simulink model "decoder"  (R2025b)
settings: Solver=VariableStepAuto  StartTime=0.0  StopTime=10.0  RelTol=1e-3
settings Model: Creator=cyber  LastModifiedBy=cyber

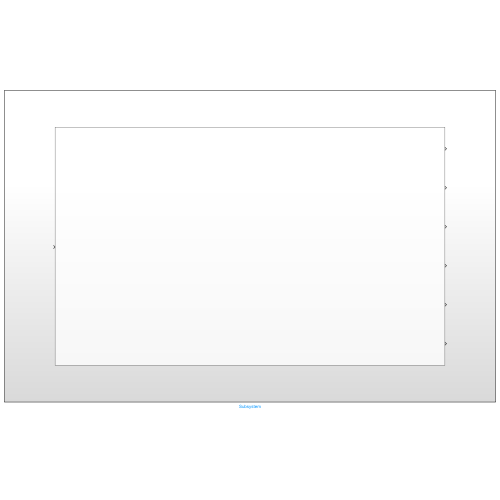
[thumbnail: Simulink's stored preview of the top-level diagram]
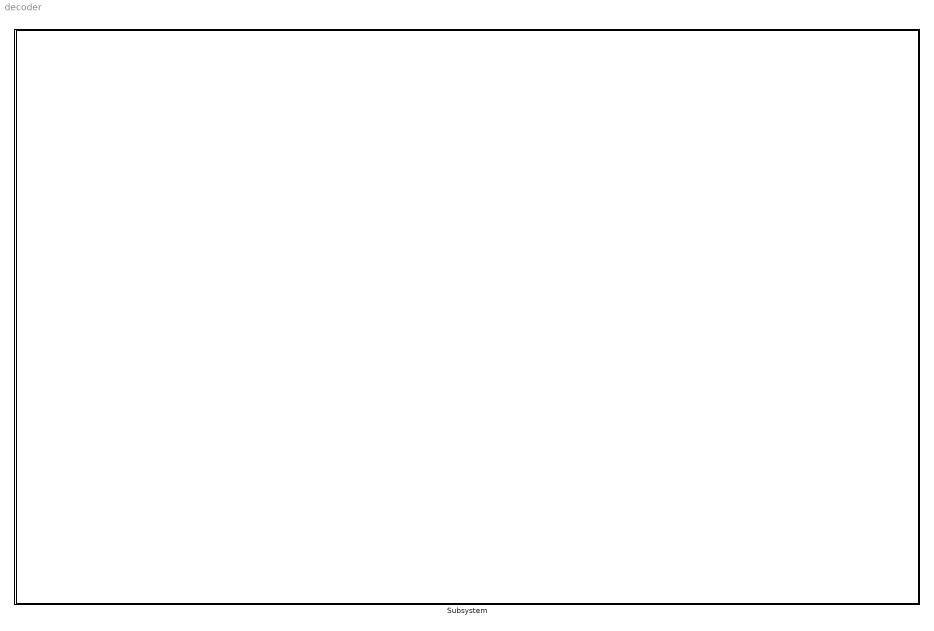
== system decoder ==
  Subsystem : Subsystem

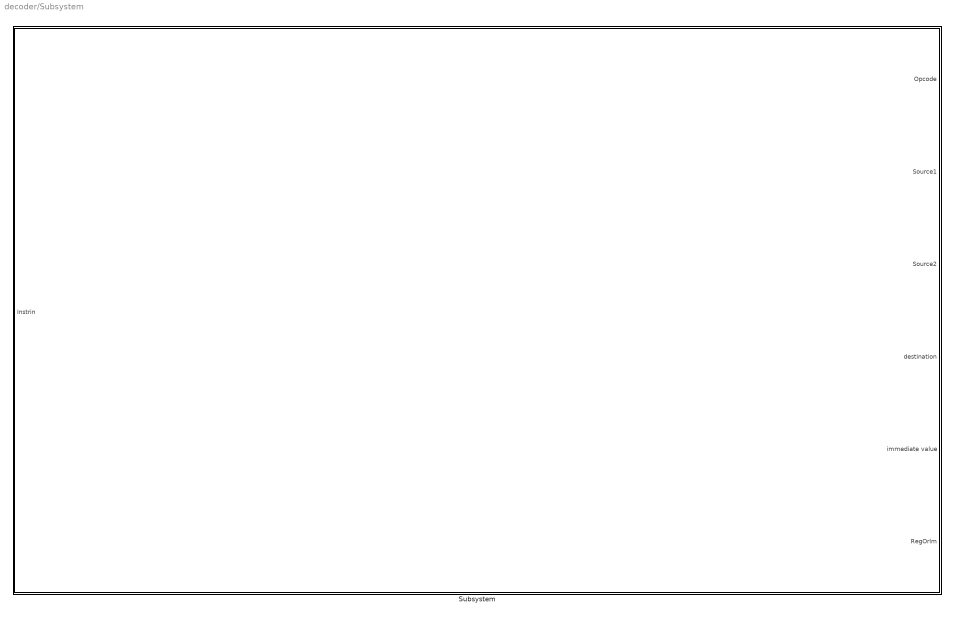
== system decoder/Subsystem ==
  Subsystem : Subsystem

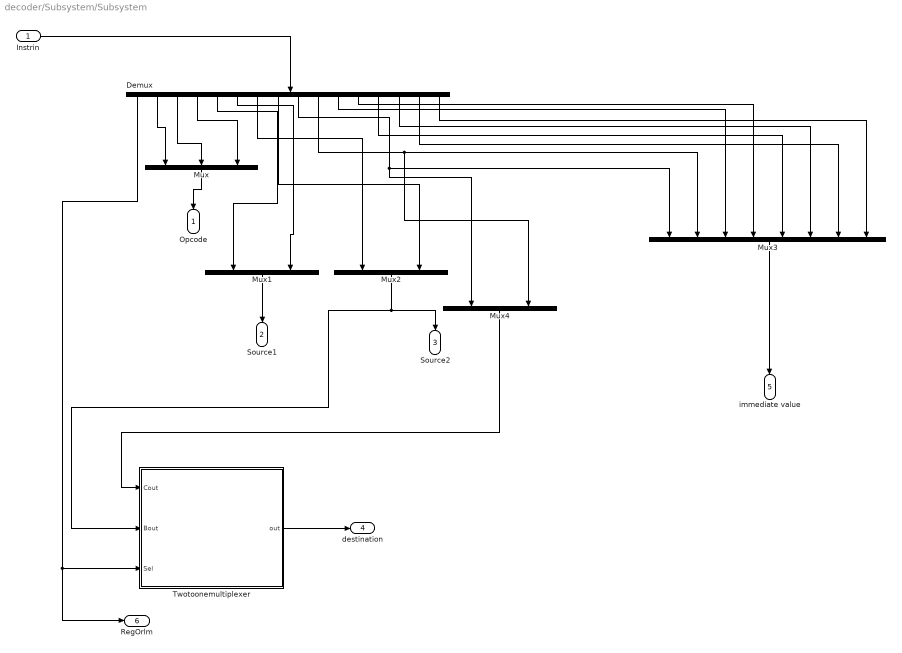
== system decoder/Subsystem/Subsystem ==
  Instrin : Inport
  Demux : Demux  Outputs=16
  Mux : Mux  Inputs=3
  Mux1 : Mux  Inputs=2
  Mux2 : Mux  Inputs=2
  Mux3 : Mux  Inputs=8
  Mux4 : Mux  Inputs=2
  Twotoonemultiplexer : Subsystem
  Opcode : Outport
  Source1 : Outport  Port=2
  Source2 : Outport  Port=3
  destination : Outport  Port=4
  immediate value : Outport  Port=5
  RegOrlm : Outport  Port=6
  wires:
  Demux/12 -> Mux3/4
  Twotoonemultiplexer/1(out) -> destination/1
  Demux/14 -> Mux3/6
  Demux/1 -> RegOrlm/1, Twotoonemultiplexer/3(Sel)
  Mux2/1 -> Source2/1, Twotoonemultiplexer/2(Bout)
  Demux/10 -> Mux4/2, Mux3/2
  Demux/16 -> Mux3/8
  Demux/9 -> Mux4/1, Mux3/1
  Demux/4 -> Mux/3
  Mux4/1 -> Twotoonemultiplexer/1(Cout)
  Demux/8 -> Mux2/2
  Demux/2 -> Mux/1
  Mux3/1 -> immediate value/1
  Demux/7 -> Mux2/1
  Demux/3 -> Mux/2
  Demux/6 -> Mux1/2
  Mux/1 -> Opcode/1
  Mux1/1 -> Source1/1
  Demux/15 -> Mux3/7
  Demux/11 -> Mux3/3
  Demux/13 -> Mux3/5
  Demux/5 -> Mux1/1
  Instrin/1 -> Demux/1

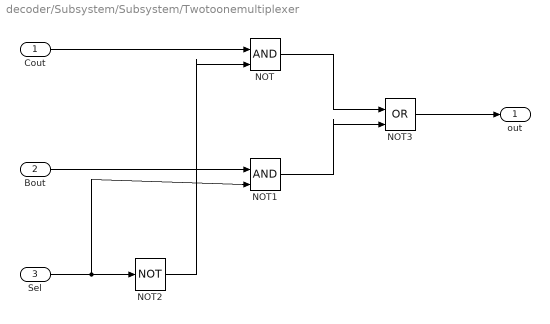
== system decoder/Subsystem/Subsystem/Twotoonemultiplexer ==
  Cout : Inport
  Bout : Inport  Port=2
  Sel : Inport  Port=3
  NOT : Logic  IconShape=distinctive  AllPortsSameDT=off  OutDataTypeStr=boolean
  NOT1 : Logic  IconShape=distinctive  AllPortsSameDT=off  OutDataTypeStr=boolean
  NOT2 : Logic  Operator=NOT  IconShape=distinctive  AllPortsSameDT=off  OutDataTypeStr=boolean
  NOT3 : Logic  Operator=OR  IconShape=distinctive  AllPortsSameDT=off  OutDataTypeStr=boolean
  out : Outport
  wires:
  Cout/1 -> NOT/1
  Sel/1 -> NOT1/2, NOT2/1
  NOT1/1 -> NOT3/2
  Bout/1 -> NOT1/1
  NOT2/1 -> NOT/2
  NOT/1 -> NOT3/1
  NOT3/1 -> out/1
